simulink model "test_hie_hot"  (R2014a)
settings: Solver=ode45  StartTime=0.0  StopTime=100  RelTol=1e-3
values from neighbouring files (symbols this model uses):
  Fa = 0.35    [HVAC_hierarchical.m]
  Fw = 0.4    [HVAC_hierarchical.m]
  tai = MAT(i+1)    [HVAC_hierarchical.m]
  twi = 100    [HVAC_hierarchical.m]
settings Model: Creator=meisu  LastModifiedBy=meisu
settings DebuggingCC: MergeDetectMultiDrivingBlocksExec=error

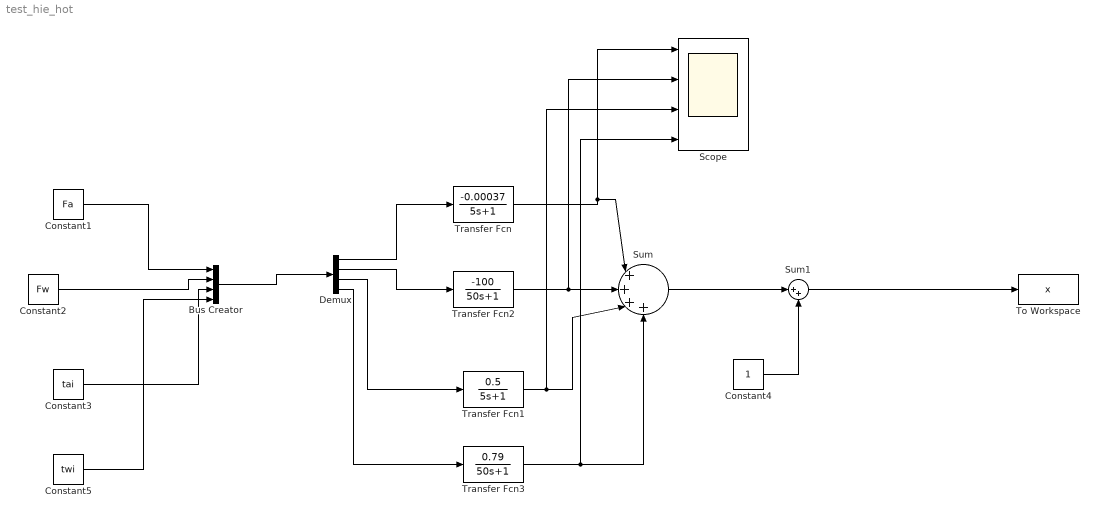
== system test_hie_hot ==
  Bus Creator : BusCreator
  Constant1 : Constant  Value=Fa
  Constant2 : Constant  Value=Fw
  Constant3 : Constant  Value=tai
  Constant4 : Constant
  Constant5 : Constant  Value=twi
  Demux : Demux
  Scope : Scope  NumInputPorts=4
      settings: YMin=-5~-5~-5~-5  YMax=5~5~5~5
  Sum : Sum  Inputs=|++++
  Sum1 : Sum  Inputs=|++
  To Workspace : ToWorkspace  VariableName=x  SaveFormat=Timeseries  SampleTime=-1
  Transfer Fcn : TransferFcn  Numerator=[-0.00037]  Denominator=[5 1]
  Transfer Fcn1 : TransferFcn  Numerator=[0.5]  Denominator=[5 1]
  Transfer Fcn2 : TransferFcn  Numerator=[-100]  Denominator=[50 1]
  Transfer Fcn3 : TransferFcn  Numerator=[0.79]  Denominator=[50 1]
  wires:
  Transfer Fcn/1 -> Scope/1, Sum/1
  Transfer Fcn2/1 -> Sum/2, Scope/2
  Transfer Fcn1/1 -> Scope/3, Sum/3
  Transfer Fcn3/1 -> Scope/4, Sum/4
  Sum/1 -> Sum1/1
  Constant4/1 -> Sum1/2
  Demux/1 -> Transfer Fcn/1
  Constant1/1 -> Bus Creator/1
  Constant2/1 -> Bus Creator/2
  Constant3/1 -> Bus Creator/3
  Demux/2 -> Transfer Fcn2/1
  Demux/3 -> Transfer Fcn1/1
  Constant5/1 -> Bus Creator/4
  Bus Creator/1 -> Demux/1
  Demux/4 -> Transfer Fcn3/1
  Sum1/1 -> To Workspace/1
